simulink subsystem "SenalizacionLuces"  (R2023b)
settings: Solver=VariableStepAuto  StartTime=0.0  StopTime=10.0  RelTol=1e-3
settings Model: Creator=Andrés  LastModifiedBy=Andrés

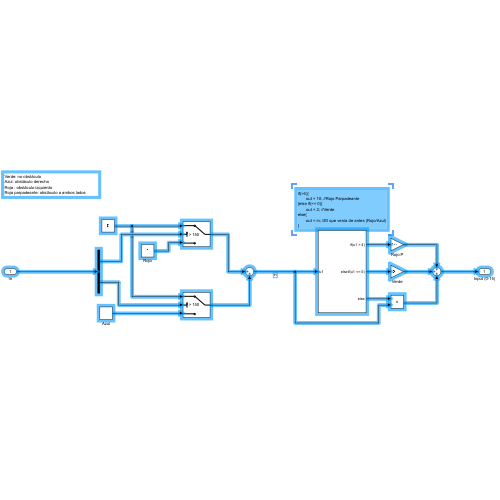
[thumbnail: Simulink's stored preview of the top-level diagram]
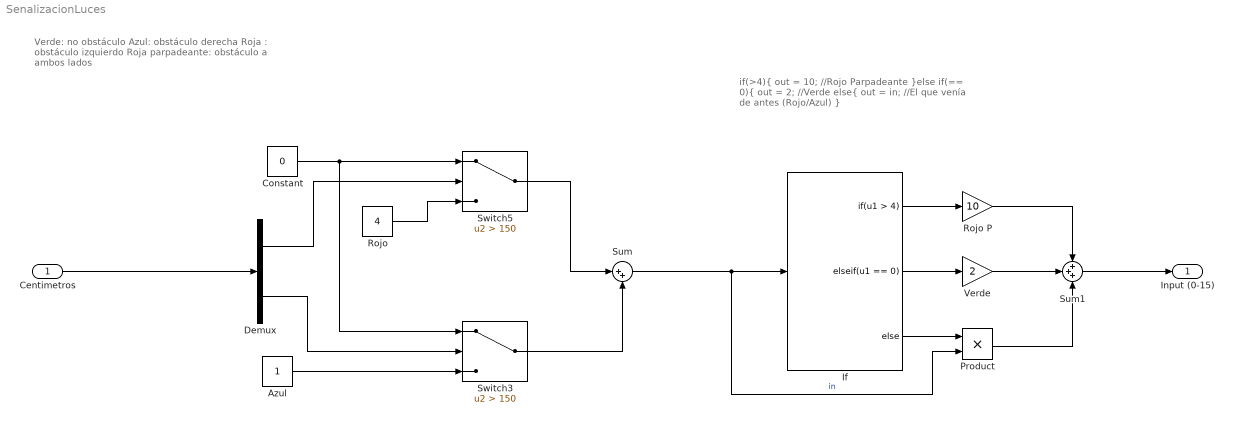
== system SenalizacionLuces ==
  note: Verde: no obstáculo
      | Azul: obstáculo derecha
      | Roja : obstáculo izquierdo
      | Roja parpadeante: obstáculo a ambos lados
  note: if(>4){
      | 	out = 10; //Rojo Parpadeante
      | }else if(== 0){
      | 	out = 2; //Verde
      | else{
      | 	out = in; //El que venía de antes (Rojo/Azul)
      | }
  Centimetros : Inport
  Azul : Constant
  Constant : Constant  Value=0
  Demux : Demux  Outputs=2
  If : If  IfExpression=u1 > 4  ElseIfExpressions=u1 == 0
  Product : Product
  Rojo : Constant  Value=4
  Rojo P : Gain  Gain=10
  Sum : Sum  Inputs=|++
  Sum1 : Sum  Inputs=+++
  Switch3 : Switch  Criteria=u2 > Threshold  Threshold=150  SaturateOnIntegerOverflow=off  InputSameDT=off
  Switch5 : Switch  Criteria=u2 > Threshold  Threshold=150  SaturateOnIntegerOverflow=off  InputSameDT=off
  Verde : Gain  Gain=2
  Input (0-15) : Outport
  wires:
  Product/1 -> Sum1/3
  Rojo P/1 -> Sum1/1
  Sum1/1 -> Input (0-15)/1
  Verde/1 -> Sum1/2
  Azul/1 -> Switch3/3
  Switch3/1 -> Sum/2
  Switch5/1 -> Sum/1
  If/3 -> Product/1
  Constant/1 -> Switch3/1, Switch5/1
  Demux/1 -> Switch5/2
  Rojo/1 -> Switch5/3
  Demux/2 -> Switch3/2
  Centimetros/1 -> Demux/1
  If/2 -> Verde/1
  Sum/1 -> Product/2, If/1  "in"
  If/1 -> Rojo P/1
